simulink library "component_lib"  (R2020b)
settings: Solver=VariableStepAuto  StartTime=0.0  StopTime=10.0  RelTol=1e-3
undefined symbols (not defined in the file or in its folder): ECCV_r, par
libraries: base_lib x70, $bdroot x59, simulink x3, pid_lib x1
(part 3 of 3)

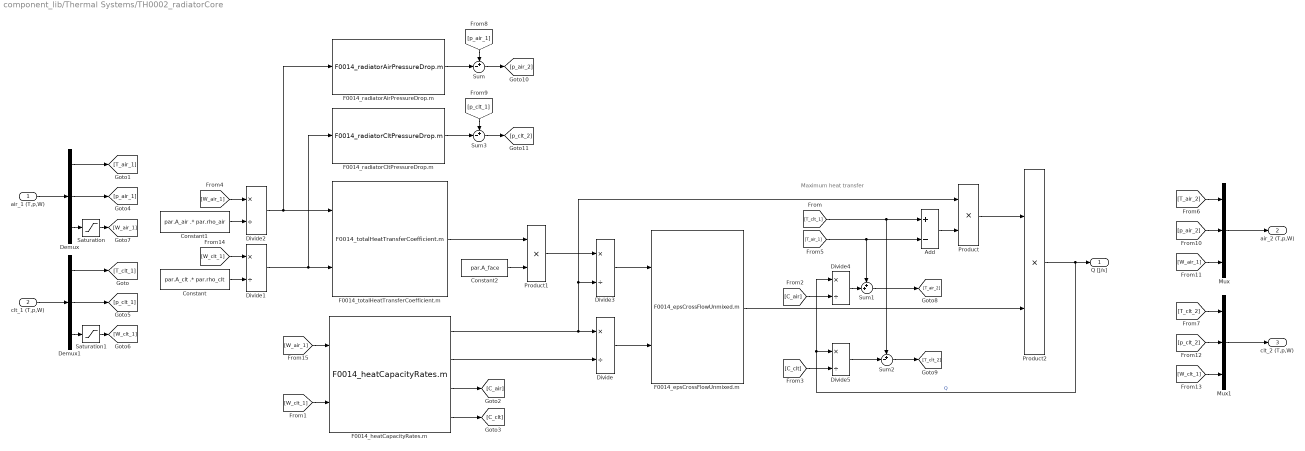
== system component_lib/Thermal Systems/TH0002_radiatorCore ==
  note: Maximum heat transfer
  air_1 (T,p,W) : Inport
  clt_1 (T,p,W) : Inport  Port=2
  Add : Sum  Inputs=+-
  Constant : Constant  Value=par.A_clt .* par.rho_clt
  Constant1 : Constant  Value=par.A_air .* par.rho_air
  Constant2 : Constant  Value=par.A_face
  Demux : Demux  Outputs=3
  Demux1 : Demux  Outputs=3
  Divide{,1..5} (6 alike) : Product  Inputs=*/
  F0014_epsCrossFlowUnmixed.m : base_lib/F0014_titanXradiator/F0014_epsCrossFlowUnmixed.m  SystemSampleTime=-1  VariantActivationTime=update diagram  Latency=0  AutoFrameSizeCalculation=off
  F0014_heatCapacityRates.m : base_lib/F0014_titanXradiator/F0014_heatCapacityRates.m  SystemSampleTime=-1  VariantActivationTime=update diagram  Latency=0  AutoFrameSizeCalculation=off
  F0014_radiatorAirPressureDrop.m : base_lib/F0014_titanXradiator/F0014_radiatorAirPressureDrop.m  SystemSampleTime=-1  VariantActivationTime=update diagram  Latency=0  AutoFrameSizeCalculation=off
  F0014_radiatorCltPressureDrop.m : base_lib/F0014_titanXradiator/F0014_radiatorCltPressureDrop.m  SystemSampleTime=-1  VariantActivationTime=update diagram  Latency=0  AutoFrameSizeCalculation=off
  F0014_totalHeatTransferCoefficient.m : base_lib/F0014_titanXradiator/F0014_totalHeatTransferCoefficient.m  SystemSampleTime=-1  VariantActivationTime=update diagram  Latency=0  AutoFrameSizeCalculation=off
  Mux : Mux  Inputs=3
  Mux1 : Mux  Inputs=3
  Product : Product
  Product1 : Product
  Product2 : Product
  Saturation : Saturate  UpperLimit=inf  LowerLimit=1e-5
  Saturation1 : Saturate  UpperLimit=inf  LowerLimit=1e-5
  Sum : Sum  Inputs=+-|
  Sum1 : Sum  Inputs=++|
  Sum2 : Sum  Inputs=+-|
  Sum3 : Sum  Inputs=+-|
  Q [J/s] : Outport
  air_2 (T,p,W) : Outport  Port=2
  clt_2 (T,p,W) : Outport  Port=3
  wires:
  F0014_heatCapacityRates.m/2 -> Divide/2
  F0014_heatCapacityRates.m/1 -> Product/1, Divide3/2, Divide/1
  Divide/1 -> F0014_epsCrossFlowUnmixed.m/2
  Constant/1 -> Divide1/2
  Divide1/1 -> F0014_radiatorCltPressureDrop.m/1, F0014_totalHeatTransferCoefficient.m/2
  [W_air_1] -> Divide2/1
  Constant1/1 -> Divide2/2
  Divide2/1 -> F0014_radiatorAirPressureDrop.m/1, F0014_totalHeatTransferCoefficient.m/1
  F0014_totalHeatTransferCoefficient.m/1 -> Product1/1
  Constant2/1 -> Product1/2
  Product1/1 -> Divide3/1
  Divide3/1 -> F0014_epsCrossFlowUnmixed.m/1
  F0014_epsCrossFlowUnmixed.m/1 -> Product2/2
  Add/1 -> Product/2
  Product2/1 -> Q [J/s]/1, Divide4/1, Divide5/1  "Q"
  [T_clt_1] -> Sum2/1, Add/1
  Product/1 -> Product2/1
  F0014_heatCapacityRates.m/3 -> [C_air]
  F0014_heatCapacityRates.m/4 -> [C_clt]
  [T_air_1] -> Add/2, Sum1/1
  Divide4/1 -> Sum1/2
  [C_air] -> Divide4/2
  [C_clt] -> Divide5/2
  Divide5/1 -> Sum2/2
  air_1 (T,p,W)/1 -> Demux/1
  clt_1 (T,p,W)/1 -> Demux1/1
  Demux1/1 -> [T_clt_1]
  Demux/1 -> [T_air_1]
  Demux/2 -> [p_air_1]
  Demux1/2 -> [p_clt_1]
  Sum1/1 -> [T_air_2]
  Sum2/1 -> [T_clt_2]
  Mux/1 -> air_2 (T,p,W)/1
  [p_air_1] -> Sum/1
  F0014_radiatorAirPressureDrop.m/1 -> Sum/2
  Sum/1 -> [p_air_2]
  Sum3/1 -> [p_clt_2]
  F0014_radiatorCltPressureDrop.m/1 -> Sum3/2
  [p_clt_1] -> Sum3/1
  [T_clt_2] -> Mux1/1
  [T_air_2] -> Mux/1
  [p_air_2] -> Mux/2
  [W_air_1] -> Mux/3
  [p_clt_2] -> Mux1/2
  [W_clt_1] -> Mux1/3
  Mux1/1 -> clt_2 (T,p,W)/1
  Demux1/3 -> Saturation1/1
  Saturation1/1 -> [W_clt_1]
  Demux/3 -> Saturation/1
  Saturation/1 -> [W_air_1]
  [W_clt_1] -> F0014_heatCapacityRates.m/2
  [W_clt_1] -> Divide1/1
  [W_air_1] -> F0014_heatCapacityRates.m/1

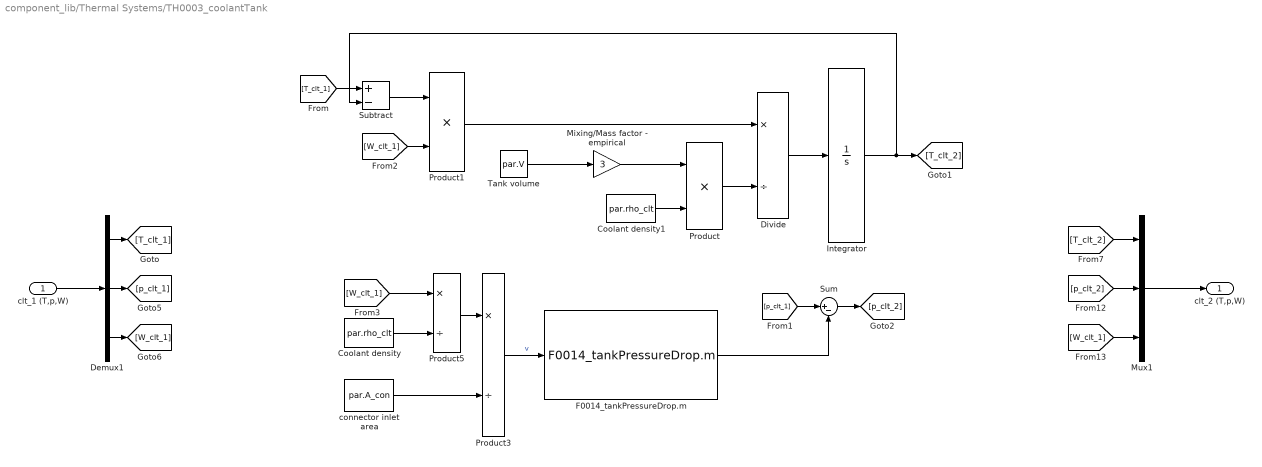
== system component_lib/Thermal Systems/TH0003_coolantTank ==
  clt_1 (T,p,W) : Inport
  Coolant density : Constant  Value=par.rho_clt
  Coolant density1 : Constant  Value=par.rho_clt
  Demux1 : Demux  Outputs=3
  Divide : Product  Inputs=*/
  F0014_tankPressureDrop.m : base_lib/F0014_titanXradiator/F0014_tankPressureDrop.m  SystemSampleTime=-1  VariantActivationTime=update diagram  Latency=0  AutoFrameSizeCalculation=off
      settings: SourceProductBaseCode=SL
  Integrator : Integrator  InitialCondition=T_0
  Mixing/Mass factor - empirical : Gain  Gain=3
  Mux1 : Mux  Inputs=3
  Product : Product
  Product1 : Product
  Product3 : Product  Inputs=*/
  Product5 : Product  Inputs=*/
  Subtract : Sum  Inputs=+-
  Sum : Sum  Inputs=|+-
  Tank volume : Constant  Value=par.V
  connector inlet area : Constant  Value=par.A_con
  clt_2 (T,p,W) : Outport
  wires:
  clt_1 (T,p,W)/1 -> Demux1/1
  Demux1/3 -> [W_clt_1]
  Demux1/1 -> [T_clt_1]
  Demux1/2 -> [p_clt_1]
  Mux1/1 -> clt_2 (T,p,W)/1
  [p_clt_2] -> Mux1/2
  [W_clt_1] -> Mux1/3
  [T_clt_2] -> Mux1/1
  Tank volume/1 -> Mixing/Mass factor - empirical/1
  [W_clt_1] -> Product5/1
  [p_clt_1] -> Sum/1
  [T_clt_1] -> Subtract/1
  [W_clt_1] -> Product1/2
  Subtract/1 -> Product1/1
  Integrator/1 -> [T_clt_2], Subtract/2
  Coolant density/1 -> Product5/2
  Mixing/Mass factor - empirical/1 -> Product/1
  Product/1 -> Divide/2
  Product1/1 -> Divide/1
  connector inlet area/1 -> Product3/2
  Sum/1 -> [p_clt_2]
  Product5/1 -> Product3/1
  Divide/1 -> Integrator/1
  F0014_tankPressureDrop.m/1 -> Sum/2
  Product3/1 -> F0014_tankPressureDrop.m/1  "v"
  Coolant density1/1 -> Product/2

== system component_lib/Thermal Systems/TH0004_radiatorPlugFlow ==
  clt_1 (T,p,W) : Inport
  Demux1 : Demux  Outputs=3
  F0014_coreFlowDelay.m : base_lib/F0014_titanXradiator/F0014_coreFlowDelay.m  SystemSampleTime=-1  VariantActivationTime=update diagram  Latency=0  AutoFrameSizeCalculation=off
  Mux1 : Mux  Inputs=3
  Saturation1 : Saturate  UpperLimit=inf  LowerLimit=1e-5
  Variable Transport Delay1 : VariableTransportDelay  VariableDelayType=Variable transport delay  MaximumDelay=20  InitialOutput=T_0  MaximumPoints=10240  TransDelayFeedthrough=on
  clt_2 (T,p,W) : Outport
  wires:
  F0014_coreFlowDelay.m/1 -> Variable Transport Delay1/2
  Variable Transport Delay1/1 -> Mux1/1
  clt_1 (T,p,W)/1 -> Demux1/1
  Demux1/3 -> Saturation1/1
  Demux1/2 -> [p_clt_1]
  Demux1/1 -> Variable Transport Delay1/1
  [p_clt_1] -> Mux1/2
  Mux1/1 -> clt_2 (T,p,W)/1
  Saturation1/1 -> Mux1/3, F0014_coreFlowDelay.m/1

== system component_lib/Thermal Systems/TH0005_flowSplit ==
  in_1 (T,p,W) : Inport
  split_fraction [-] : Inport  Port=2
  Demux1 : Demux  Outputs=3
  Mux1 : Mux  Inputs=3
  Mux2 : Mux  Inputs=3
  Product : Product
  Sum : Sum  Inputs=-+|
  out_21 (T,p,W) : Outport
  out_22 (T,p,W) : Outport  Port=2
  wires:
  Product/1 -> Mux1/3, Sum/1
  in_1 (T,p,W)/1 -> Demux1/1
  Demux1/3 -> Sum/2, Product/1
  Mux1/1 -> out_21 (T,p,W)/1
  split_fraction [-]/1 -> Product/2
  Mux2/1 -> out_22 (T,p,W)/1
  Sum/1 -> Mux2/3
  Demux1/1 -> [T_1]
  Demux1/2 -> Mux2/2, Mux1/2
  [T_1] -> Mux1/1
  [T_1] -> Mux2/1

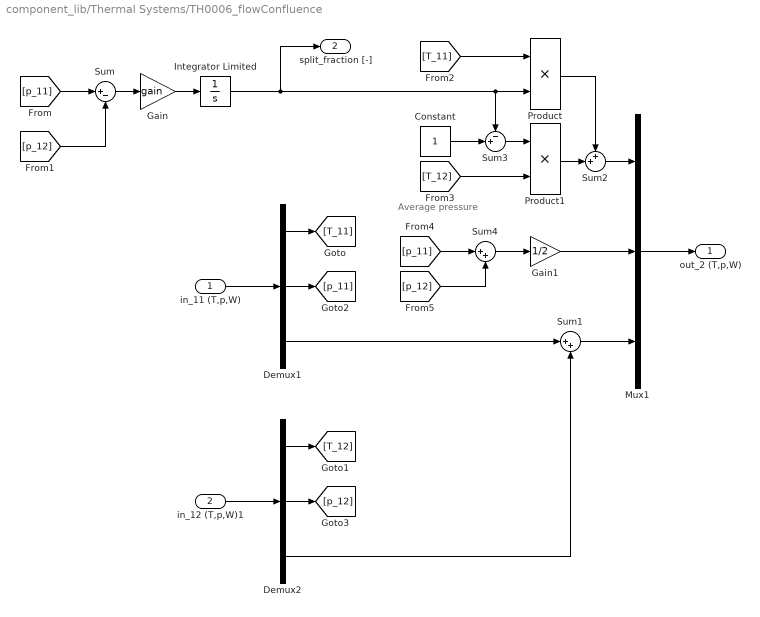
== system component_lib/Thermal Systems/TH0006_flowConfluence ==
  note: Average pressure
  in_11 (T,p,W) : Inport
  in_12 (T,p,W)1 : Inport  Port=2
  Constant : Constant
  Demux1 : Demux  Outputs=3
  Demux2 : Demux  Outputs=3
  Gain : Gain  Gain=gain
  Gain1 : Gain  Gain=1/2
  Integrator Limited : Integrator  InitialCondition=0.5  LimitOutput=on  UpperSaturationLimit=1  LowerSaturationLimit=0
  Mux1 : Mux  Inputs=3
  Product : Product
  Product1 : Product
  Sum : Sum  Inputs=|+-
  Sum1 : Sum  Inputs=|++
  Sum2 : Sum  Inputs=++|
  Sum3 : Sum  Inputs=-+|
  Sum4 : Sum  Inputs=|++
  out_2 (T,p,W) : Outport
  split_fraction [-] : Outport  Port=2
  wires:
  in_11 (T,p,W)/1 -> Demux1/1
  Mux1/1 -> out_2 (T,p,W)/1
  in_12 (T,p,W)1/1 -> Demux2/1
  Sum/1 -> Gain/1
  Gain/1 -> Integrator Limited/1
  Integrator Limited/1 -> split_fraction [-]/1, Product/2, Sum3/1
  Demux1/1 -> [T_11]
  Demux2/1 -> [T_12]
  Demux1/3 -> Sum1/1
  Sum1/1 -> Mux1/3
  Demux2/3 -> Sum1/2
  Demux1/2 -> [p_11]
  Demux2/2 -> [p_12]
  [p_11] -> Sum/1
  [p_12] -> Sum/2
  [T_11] -> Product/1
  Product/1 -> Sum2/1
  Product1/1 -> Sum2/2
  Sum2/1 -> Mux1/1
  Constant/1 -> Sum3/2
  [p_11] -> Sum4/1
  Sum4/1 -> Gain1/1
  [p_12] -> Sum4/2
  Gain1/1 -> Mux1/2
  Sum3/1 -> Product1/1
  [T_12] -> Product1/2

== system component_lib/Thermal Systems/TH0007_airRestriction ==
  air_1 (T,p,W) : Inport
  Demux1 : Demux  Outputs=3
  F0014_restrictionPressureDrop.m : base_lib/F0014_titanXradiator/F0014_restrictionPressureDrop.m  SystemSampleTime=-1  VariantActivationTime=update diagram  Latency=0  AutoFrameSizeCalculation=off
      settings: SourceProductBaseCode=SL
  Mux1 : Mux  Inputs=3
  Sum : Sum  Inputs=-+|
  air_2 (T,p,W) : Outport
  wires:
  Mux1/1 -> air_2 (T,p,W)/1
  air_1 (T,p,W)/1 -> Demux1/1
  Demux1/3 -> Mux1/3, F0014_restrictionPressureDrop.m/3
  Demux1/1 -> F0014_restrictionPressureDrop.m/1, Mux1/1
  F0014_restrictionPressureDrop.m/1 -> Sum/1
  Sum/1 -> Mux1/2
  Demux1/2 -> F0014_restrictionPressureDrop.m/2, Sum/2

== system component_lib/Thermal Systems/TH0008_condenser ==
  air_1 (T,p,W) : Inport
  Q [J/s] : Inport  Port=2
  AIrCp : Constant  Value=par.cp_air
  Demux1 : Demux  Outputs=3
  F0014_condenserPressureDrop.m : base_lib/F0014_titanXradiator/F0014_condenserPressureDrop.m  SystemSampleTime=-1  VariantActivationTime=update diagram  Latency=0  AutoFrameSizeCalculation=off
  Mux1 : Mux  Inputs=3
  Product3 : Product  Inputs=*//
  Saturation : Saturate  UpperLimit=inf  LowerLimit=0.001
  Saturation1 : Saturate  UpperLimit=373  LowerLimit=0
  Sum : Sum  Inputs=|+-
  Sum1 : Sum  Inputs=++|
  air_2 (T,p,W) : Outport
  wires:
  air_1 (T,p,W)/1 -> Demux1/1
  Mux1/1 -> air_2 (T,p,W)/1
  Q [J/s]/1 -> Product3/1
  AIrCp/1 -> Product3/3
  Product3/1 -> Sum1/2  "dT"
  Demux1/1 -> [T_1]
  Saturation/1 -> Product3/2
  Demux1/3 -> Mux1/3, F0014_condenserPressureDrop.m/3, Saturation/1
  Sum1/1 -> Saturation1/1
  Saturation1/1 -> Mux1/1
  Demux1/2 -> [p_1]
  [p_1] -> F0014_condenserPressureDrop.m/2
  [T_1] -> F0014_condenserPressureDrop.m/1
  [p_1] -> Sum/1
  Sum/1 -> Mux1/2
  F0014_condenserPressureDrop.m/1 -> Sum/2
  [T_1] -> Sum1/1

== system component_lib/Thermal Systems/TH0009_intake ==
  air_1 (T,p,W) : Inport
  v [m/s] : Inport  Port=2
  Demux1 : Demux  Outputs=3
  F0014_intakePressureIncrease.m : base_lib/F0014_titanXradiator/F0014_intakePressureIncrease.m  SystemSampleTime=-1  VariantActivationTime=update diagram  Latency=0  AutoFrameSizeCalculation=off
  Mux1 : Mux  Inputs=3
  Saturation : Saturate  UpperLimit=inf  LowerLimit=0
  Sum : Sum  Inputs=++|
  air_2 (T,p,W) : Outport
  wires:
  Mux1/1 -> air_2 (T,p,W)/1
  air_1 (T,p,W)/1 -> Demux1/1
  Sum/1 -> Mux1/2
  Demux1/2 -> Sum/2, F0014_intakePressureIncrease.m/2
  F0014_intakePressureIncrease.m/1 -> Sum/1
  Demux1/3 -> Mux1/3
  Demux1/1 -> Mux1/1, F0014_intakePressureIncrease.m/1
  v [m/s]/1 -> Saturation/1
  Saturation/1 -> F0014_intakePressureIncrease.m/3

== system component_lib/Thermal Systems/TH0010_fan ==
  note: Density
  air_1 (T,p,W) : Inport
  rel_speed [-] : Inport  Port=2
  Constant : Constant  Value=286
  Constant1 : Constant  Value=par.n_fan
  Constant2 : Constant  Value=par.dp0
  Constant3 : Constant  Value=3
  Constant4 : Constant  Value=par.P_nom
  Constant5 : Constant  Value=par.n_fan
  Demux1 : Demux  Outputs=3
  Divide : Product  Inputs=*//
  Divide1 : Product  Inputs=*//
  Divide2 : Product  Inputs=*/
  F0014_fanCurve.m : base_lib/F0014_titanXradiator/F0014_fanCurve.m  SystemSampleTime=-1  VariantActivationTime=update diagram  Latency=0  AutoFrameSizeCalculation=off
  Math Function : Math  Operator=square  SaturateOnIntegerOverflow=on
  Math Function1 : Math  Operator=pow  SaturateOnIntegerOverflow=on
  Mux : Mux  Inputs=3
  Product : Product
  Product1 : Product
  Product2 : Product  Inputs=3
  Ref. density : Constant  Value=1.18
  Sum : Sum  Inputs=|++
  Transfer Fcn : TransferFcn  Denominator=[0.1 1]
  air_2 (T,p,W) : Outport
  P_fan [J/s] : Outport  Port=2
  wires:
  air_1 (T,p,W)/1 -> Demux1/1
  Mux/1 -> air_2 (T,p,W)/1
  Demux1/3 -> Mux/3, Divide/1
  Demux1/1 -> Mux/1, [T_1]
  [T_1] -> Divide1/2
  Constant/1 -> Divide1/3
  Divide1/1 -> Divide2/1, Divide/3
  Constant1/1 -> Divide/2
  Math Function/1 -> Product/1
  Constant2/1 -> Product/2
  Divide/1 -> F0014_fanCurve.m/1
  Product/1 -> F0014_fanCurve.m/2
  F0014_fanCurve.m/1 -> Product1/1
  Ref. density/1 -> Divide2/2
  Divide2/1 -> Product1/2
  Demux1/2 -> [p_1], Sum/1
  Product1/1 -> Sum/2
  Sum/1 -> Mux/2
  [p_1] -> Divide1/1
  Transfer Fcn/1 -> Math Function/1, Math Function1/1
  rel_speed [-]/1 -> Transfer Fcn/1
  Constant3/1 -> Math Function1/2
  Math Function1/1 -> Product2/1
  Constant4/1 -> Product2/2
  Product2/1 -> P_fan [J/s]/1
  Constant5/1 -> Product2/3

== system component_lib/Thermal Systems/TH0011_coolingChannel ==
  T_w [K] : Inport
  clt_1 (T,p,W) : Inport  Port=2
  Demux : Demux  Outputs=3
  F0017_Nusselt.m : base_lib/F0017_channelCooling/F0017_Nusselt.m  SystemSampleTime=-1  VariantActivationTime=update diagram  Latency=0  AutoFrameSizeCalculation=off
      settings: SourceProductBaseCode=SL
  F0017_Prandtl.m : base_lib/F0017_channelCooling/F0017_Prandtl.m  SystemSampleTime=-1  VariantActivationTime=update diagram  Latency=0  AutoFrameSizeCalculation=off
      settings: SourceProductBaseCode=SL
  F0017_Reynolds.m : base_lib/F0017_channelCooling/F0017_Reynolds.m  SystemSampleTime=-1  VariantActivationTime=update diagram  Latency=0  AutoFrameSizeCalculation=off
      settings: SourceProductBaseCode=SL
  F0017_heatTransfer.m : base_lib/F0017_channelCooling/F0017_heatTransfer.m  SystemSampleTime=-1  VariantActivationTime=update diagram  Latency=0  AutoFrameSizeCalculation=off
      settings: SourceProductBaseCode=SL
  F0017_pressureDrop.m : base_lib/F0017_channelCooling/F0017_pressureDrop.m  SystemSampleTime=-1  VariantActivationTime=update diagram  Latency=0  AutoFrameSizeCalculation=off
      settings: SourceProductBaseCode=SL
  F0017_velocity.m : base_lib/F0017_channelCooling/F0017_velocity.m  SystemSampleTime=-1  VariantActivationTime=update diagram  Latency=0  AutoFrameSizeCalculation=off
      settings: SourceProductBaseCode=SL
  Gain : Gain  Gain=1/n_ch
  Gain1 : Gain  Gain=n_ch
  Gain2 : Gain  Gain=n_ch
  Mux : Mux  Inputs=3
  Sum : Sum  Inputs=-+|
  Q [J/s] : Outport
  clt_2 (T,p,W) : Outport  Port=2
  wires:
  clt_1 (T,p,W)/1 -> Demux/1
  Mux/1 -> clt_2 (T,p,W)/1
  F0017_velocity.m/1 -> F0017_Reynolds.m/1, F0017_pressureDrop.m/1
  F0017_Reynolds.m/1 -> F0017_pressureDrop.m/2, F0017_Nusselt.m/1
  F0017_Prandtl.m/1 -> F0017_Nusselt.m/2
  Demux/1 -> F0017_heatTransfer.m/1
  T_w [K]/1 -> F0017_heatTransfer.m/2
  F0017_Nusselt.m/1 -> F0017_heatTransfer.m/3
  Sum/1 -> [p_2]
  [p_2] -> Mux/2
  Demux/2 -> Sum/2
  Demux/3 -> Gain/1
  F0017_pressureDrop.m/1 -> Sum/1
  F0017_heatTransfer.m/1 -> Gain2/1
  F0017_heatTransfer.m/2 -> Mux/1
  Gain/1 -> F0017_velocity.m/1, Gain1/1, F0017_heatTransfer.m/4
  Gain1/1 -> Mux/3
  Gain2/1 -> Q [J/s]/1

== system component_lib/Thermal Systems/TH0011_outletFlowBalance ==
  air_1 (T,p,W) : Inport
  p_amb [Pa] : Inport  Port=2
  Demux : Demux  Outputs=3
  Gain : Gain  Gain=gain
  Integrator Limited : Integrator  LimitOutput=on  LowerSaturationLimit=0
  Sum : Sum  Inputs=|+-
  Terminator : Terminator
  Terminator1 : Terminator
  W_inlet [kg/s] : Outport
  wires:
  air_1 (T,p,W)/1 -> Demux/1
  Demux/2 -> Sum/1
  p_amb [Pa]/1 -> Sum/2
  Sum/1 -> Gain/1
  Gain/1 -> Integrator Limited/1
  Integrator Limited/1 -> W_inlet [kg/s]/1
  Demux/1 -> Terminator/1
  Demux/3 -> Terminator1/1

== system component_lib/Thermal Systems/TH0011_pipe ==
  clt_1 (T,p,W) : Inport
  Constant : Constant  Value=par.L
  Demux : Demux  Outputs=3
  Divide : Product  Inputs=*/
  F0017_Reynolds.m : base_lib/F0017_channelCooling/F0017_Reynolds.m  SystemSampleTime=-1  VariantActivationTime=update diagram  Latency=0  AutoFrameSizeCalculation=off
      settings: SourceProductBaseCode=SL
  F0017_pressureDrop.m : base_lib/F0017_channelCooling/F0017_pressureDrop.m  SystemSampleTime=-1  VariantActivationTime=update diagram  Latency=0  AutoFrameSizeCalculation=off
      settings: SourceProductBaseCode=SL
  F0017_velocity.m : base_lib/F0017_channelCooling/F0017_velocity.m  SystemSampleTime=-1  VariantActivationTime=update diagram  Latency=0  AutoFrameSizeCalculation=off
      settings: SourceProductBaseCode=SL
  Mux : Mux  Inputs=3
  Saturation : Saturate  UpperLimit=10  LowerLimit=0
  Sum : Sum  Inputs=|+-
  Variable Transport Delay : VariableTransportDelay  VariableDelayType=Variable transport delay  MaximumDelay=10  InitialOutput=T_0
  clt_2 (T,p,W) : Outport
  wires:
  clt_1 (T,p,W)/1 -> Demux/1
  Constant/1 -> Divide/1
  F0017_velocity.m/1 -> F0017_Reynolds.m/1, Divide/2, F0017_pressureDrop.m/1
  Divide/1 -> Saturation/1
  Demux/1 -> Variable Transport Delay/1
  F0017_Reynolds.m/1 -> F0017_pressureDrop.m/2
  F0017_pressureDrop.m/1 -> Sum/2
  Saturation/1 -> Variable Transport Delay/2
  Variable Transport Delay/1 -> Mux/1
  Sum/1 -> Mux/2
  Mux/1 -> clt_2 (T,p,W)/1
  Demux/3 -> Mux/3, F0017_velocity.m/1
  Demux/2 -> Sum/1

== system component_lib/Thermal Systems/TH0011_thermalMass ==
  dQ [J/s] : Inport
  Constant : Constant  Value=m
  Constant1 : Constant  Value=cp
  Integrator : Integrator  InitialCondition=T_0
  Product : Product  Inputs=*//
  T [K] : Outport
  wires:
  Integrator/1 -> T [K]/1
  Product/1 -> Integrator/1
  dQ [J/s]/1 -> Product/1
  Constant/1 -> Product/2
  Constant1/1 -> Product/3

== system component_lib/Thermal Systems/TH0012_equalSplitMerge ==
  note: merge/distribute flow
  clt_1 (T,p,W) : Inport
  Demux : Demux  Outputs=3
  Gain : Gain  Gain=n
  Mux : Mux  Inputs=3
  clt_2 (T,p,W) : Outport
  wires:
  clt_1 (T,p,W)/1 -> Demux/1
  Demux/3 -> Gain/1
  Demux/1 -> Mux/1
  Gain/1 -> Mux/3
  Demux/2 -> Mux/2
  Mux/1 -> clt_2 (T,p,W)/1

== system component_lib/Thermal Systems/TH0013_tank ==
  amb (T,p,RH) : Inport
  W_pump [kg/s] : Inport  Port=2
  p_pump [Pa] : Inport  Port=3
  clt_1 (T,p,W) : Inport  Port=4
  Constant : Constant  Value=par.cv_clt
  Constant1 : Constant  Value=par.cv_clt
  Demux : Demux  Outputs=3
  Demux1 : Demux  Outputs=3
  Divide : Product  Inputs=*//
  Divide1 : Product  Inputs=***
  F0017_temperatureToEnthalpy.m : base_lib/F0017_channelCooling/F0017_temperatureToEnthalpy.m  SystemSampleTime=-1  VariantActivationTime=update diagram  Latency=0  AutoFrameSizeCalculation=off
      settings: SourceProductBaseCode=SL
  F0017_temperatureToEnthalpy.m1 : base_lib/F0017_channelCooling/F0017_temperatureToEnthalpy.m  SystemSampleTime=-1  VariantActivationTime=update diagram  Latency=0  AutoFrameSizeCalculation=off
      settings: SourceProductBaseCode=SL
  Integrator : Integrator  InitialCondition=V .* par.rho_clt  LimitOutput=on  LowerSaturationLimit=1e-3
  Integrator1 : Integrator  InitialConditionSource=external  InitialCondition=293  LimitOutput=on  LowerSaturationLimit=1e-3
  Mux : Mux  Inputs=3
  Product : Product
  Product1 : Product
  Sum : Sum  Inputs=+|-
  Sum2 : Sum  Inputs=+--
  Sum3 : Sum  Inputs=|-+
  Terminator : Terminator
  m_clt [kg] : Outport
  clt_2 (T,p,W) : Outport  Port=2
  wires:
  clt_1 (T,p,W)/1 -> Demux/1
  Mux/1 -> clt_2 (T,p,W)/1
  Sum/1 -> Divide1/3, Integrator/1
  Demux/3 -> Product/2, Sum/1
  Integrator/1 -> m_clt [kg]/1, Divide/3
  p_pump [Pa]/1 -> Mux/2
  Demux/2 -> Terminator/1
  Demux/1 -> F0017_temperatureToEnthalpy.m/1, [T_1]
  F0017_temperatureToEnthalpy.m/1 -> Product/1
  F0017_temperatureToEnthalpy.m1/1 -> Product1/1
  Integrator1/1 -> F0017_temperatureToEnthalpy.m1/1, Sum3/2, Mux/1
  Constant/1 -> Divide/2
  W_pump [kg/s]/1 -> Product1/2, Mux/3, Sum/2
  [T_1] -> Sum3/1
  Sum3/1 -> Divide1/2
  Sum2/1 -> Divide/1
  Divide1/1 -> Sum2/2
  Divide/1 -> Integrator1/1
  Constant1/1 -> Divide1/1
  Product/1 -> Sum2/1
  Product1/1 -> Sum2/3
  amb (T,p,RH)/1 -> Demux1/1
  Demux1/1 -> Integrator1/2

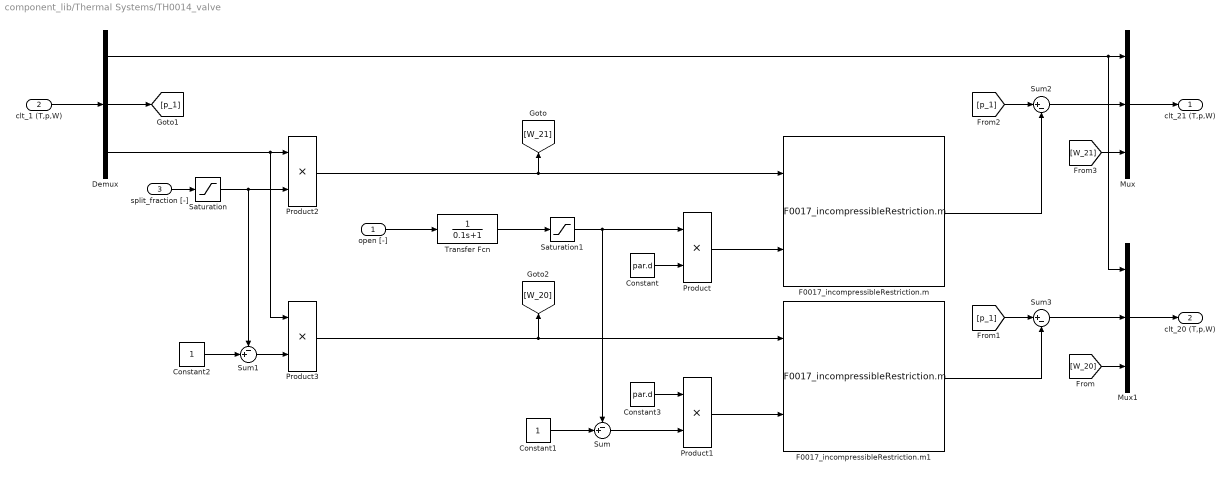
== system component_lib/Thermal Systems/TH0014_valve ==
  open [-] : Inport
  clt_1 (T,p,W) : Inport  Port=2
  split_fraction [-] : Inport  Port=3
  Constant : Constant  Value=par.d
  Constant1 : Constant
  Constant2 : Constant
  Constant3 : Constant  Value=par.d
  Demux : Demux  Outputs=3
  F0017_incompressibleRestriction.m : base_lib/F0017_channelCooling/F0017_incompressibleRestriction.m  SystemSampleTime=-1  VariantActivationTime=update diagram  Latency=0  AutoFrameSizeCalculation=off
      settings: SourceProductBaseCode=SL
  F0017_incompressibleRestriction.m1 : base_lib/F0017_channelCooling/F0017_incompressibleRestriction.m  SystemSampleTime=-1  VariantActivationTime=update diagram  Latency=0  AutoFrameSizeCalculation=off
      settings: SourceProductBaseCode=SL
  Mux : Mux  Inputs=3
  Mux1 : Mux  Inputs=3
  Product{,1..3} (4 alike) : Product
  Saturation : Saturate  UpperLimit=1  LowerLimit=0
  Saturation1 : Saturate  UpperLimit=0.99  LowerLimit=0.01
  Sum : Sum  Inputs=-+|
  Sum1 : Sum  Inputs=-+|
  Sum2 : Sum  Inputs=|+-
  Sum3 : Sum  Inputs=|+-
  Transfer Fcn : TransferFcn  Denominator=[0.1 1]
  clt_21 (T,p,W) : Outport
  clt_20 (T,p,W) : Outport  Port=2
  wires:
  clt_1 (T,p,W)/1 -> Demux/1
  Mux/1 -> clt_21 (T,p,W)/1
  Saturation1/1 -> Sum/1, Product/1
  Constant1/1 -> Sum/2
  Sum/1 -> Product1/2
  Constant2/1 -> Sum1/2
  Product2/1 -> F0017_incompressibleRestriction.m/1, [W_21]
  Product3/1 -> F0017_incompressibleRestriction.m1/1, [W_20]
  Sum1/1 -> Product3/2
  Demux/3 -> Product3/1, Product2/1
  Mux1/1 -> clt_20 (T,p,W)/1
  Sum2/1 -> Mux/2
  F0017_incompressibleRestriction.m/1 -> Sum2/2
  Demux/1 -> Mux1/1, Mux/1
  [W_20] -> Mux1/3
  Demux/2 -> [p_1]
  Sum3/1 -> Mux1/2
  [p_1] -> Sum3/1
  F0017_incompressibleRestriction.m1/1 -> Sum3/2
  [p_1] -> Sum2/1
  [W_21] -> Mux/3
  Saturation/1 -> Sum1/1, Product2/2
  split_fraction [-]/1 -> Saturation/1
  open [-]/1 -> Transfer Fcn/1
  Transfer Fcn/1 -> Saturation1/1
  Constant/1 -> Product/2
  Constant3/1 -> Product1/1
  Product/1 -> F0017_incompressibleRestriction.m/2
  Product1/1 -> F0017_incompressibleRestriction.m1/2

== system component_lib/Thermal Systems/TH0015_totalHeatTransfer ==
  Q [J/s] : Inport
  clt_1 (T,p,W) : Inport  Port=2
  Constant : Constant  Value=par.cp_clt
  Demux : Demux  Outputs=3
  Mux : Mux  Inputs=3
  Product : Product  Inputs=*//
  Sum : Sum  Inputs=++|
  clt_2 (T,p,W) : Outport
  wires:
  clt_1 (T,p,W)/1 -> Demux/1
  Mux/1 -> clt_2 (T,p,W)/1
  Demux/3 -> Mux/3, Product/2
  Demux/2 -> Mux/2
  Sum/1 -> Mux/1
  Q [J/s]/1 -> Product/1
  Constant/1 -> Product/3
  Demux/1 -> Sum/2
  Product/1 -> Sum/1
